simulink model "sgp4_unit_test"  (R2016b)
settings: Solver=FixedStepAuto  StartTime=0.0  StopTime=259200  RelTol=1e-3
values from neighbouring files (symbols this model uses):
  fsw_params = init_fsw_params()    [sgp4_test_init.m]
libraries: time_conversion_lib x1, MET_lib x1, sgp4_lib_fsw x1, time_coord_rotation_lib x1
settings Model: SimulationMode=accelerator  Creator=taylorreynolds  LastModifiedBy=Taylor

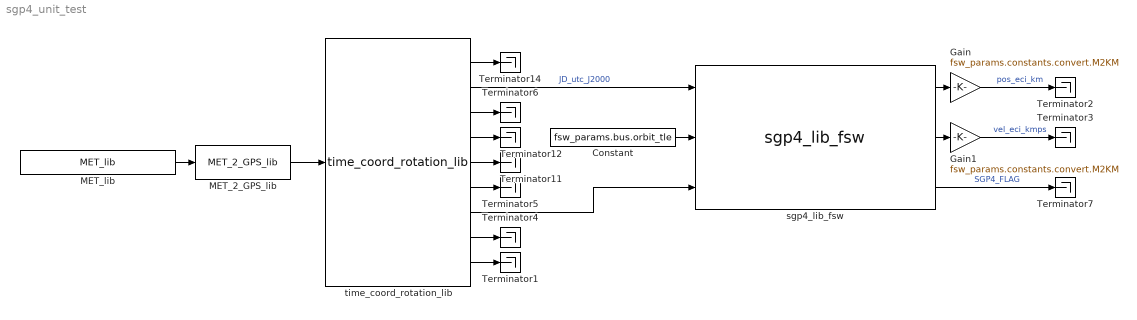
== system sgp4_unit_test ==
  Constant : Constant  Value=fsw_params.bus.orbit_tle
  Gain : Gain  Gain=fsw_params.constants.convert.M2KM
  Gain1 : Gain  Gain=fsw_params.constants.convert.M2KM
  MET_2_GPS_lib : time_conversion_lib/MET_2_GPS_lib
  MET_lib : MET_lib/MET_lib
  Terminator{1..7,11..12,14} (10 alike) : Terminator
  sgp4_lib_fsw : sgp4_lib_fsw/sgp4_lib_fsw
  time_coord_rotation_lib : time_coord_rotation_lib/time_coord_rotation_lib
  wires:
  Gain/1 -> Terminator2/1  "pos_eci_km"
  Gain1/1 -> Terminator3/1  "vel_eci_kmps"
  Constant/1 -> sgp4_lib_fsw/2
  time_coord_rotation_lib/6 -> Terminator5/1
  time_coord_rotation_lib/8 -> Terminator4/1
  time_coord_rotation_lib/5 -> Terminator11/1
  time_coord_rotation_lib/4 -> Terminator12/1
  time_coord_rotation_lib/2 -> sgp4_lib_fsw/1  "JD_utc_J2000"
  time_coord_rotation_lib/1 -> Terminator14/1
  time_coord_rotation_lib/7 -> sgp4_lib_fsw/3
  time_coord_rotation_lib/9 -> Terminator1/1
  time_coord_rotation_lib/3 -> Terminator6/1
  sgp4_lib_fsw/1 -> Gain/1
  sgp4_lib_fsw/2 -> Gain1/1
  sgp4_lib_fsw/3 -> Terminator7/1  "SGP4_FLAG"
  MET_lib/1 -> MET_2_GPS_lib/1
  MET_2_GPS_lib/1 -> time_coord_rotation_lib/1
